simulink model "UIOwDAC_balas_01"  (R2019b)
settings: Solver=VariableStepAuto  StartTime=0.0  StopTime=60  RelTol=1e-3
values from neighbouring files (symbols this model uses):
  A = A-0.1*eye(2)    [DAC_UIO_Comp.m]    (also in LinearND_QUANTUM_2020_11_14_2.m = A+(basis{i}*rand()); UIO_adaptive_example.m = [-2379.2 0 0 0 0;0 -2.3 0 0.21 0; UIO_adaptive_example_2.m = [-1/Ta, (alpha+sigma2*wb2)/Ta, (-kb*sigma2*wb2)/Ta, -kb*sigm; UIO_adaptive_example_EEG_Balas_2ch.m = A-0.4*eye(2))
  Am = double(subs(Am_sys,{ep,Lx},{0.1,1-2*j}))    [DAC_UIO_Comp.m]    (also in UIO_adaptive_example_EEG_Balas_2ch.m = [0 1;-5 -4]; UIO_adaptive_example_alternative_EEG_ch6.m = ss_c.A; UIO_alternative_2021_01_26.m = Am-.1*eye(2); UIO_alternative_PAPER_2021_02_17.m = [0 1;-1 -1])
  B = [0;1]    [DAC_UIO_Comp.m]    (also in UIO_adaptive_example_EEG_Balas_2ch.m; UIO_adaptive_example_alternative_EEG_ch6.m = ones(opt_order,1); UIO_alternative_2021_01_26.m; UIO_alternative_PAPER_2021_02_17.m = [1;0;-1])
  C = double(subs(C_sym,{ep},{0.1}))    [DAC_UIO_Comp.m]    (also in UIO_adaptive_example.m = [1 0 0 0 0;0 0 0 1 0; 0 0 0 0 1]; UIO_adaptive_example_2.m = [1 0 0 0;0 1 0 0]; UIO_adaptive_example_EEG_Balas_2ch.m = [1, epsilon]; UIO_adaptive_example_alternative_EEG_ch6.m = ss_c.C)
  g1 = 4+2j    [DAC_UIO_Comp.m]    (also in UIO_adaptive_example_EEG_Balas_2ch.m = 4; UIO_alternative_2021_01_26.m = 2+1j; UIO_alternative_PAPER_2021_02_17.m = 2; UIO_alternative_PAPER_2021_03_01.m = 2)
  g2 = 0    [DAC_UIO_Comp.m]    (also in UIO_adaptive_example_EEG_Balas_2ch.m = -0.3; UIO_alternative_2021_01_26.m; UIO_alternative_PAPER_2021_02_17.m = 1; UIO_alternative_PAPER_2021_03_01.m)
  g3 = 0    [DAC_UIO_Comp.m]    (also in UIO_adaptive_example_EEG_Balas_2ch.m = 0.1; UIO_alternative_2021_01_26.m; UIO_alternative_PAPER_2021_02_17.m = -3; UIO_alternative_PAPER_2021_03_01.m)
  gamma_e = 1    [DAC_UIO_Comp.m]    (also in UIO_adaptive_example_EEG_Balas_2ch.m; UIO_adaptive_example_alternative_EEG_ch6.m = .0001*ones(length(Am),1); UIO_alternative_2021_01_26.m = 0.001; UIO_alternative_PAPER_2021_02_17.m = 0.0001)
  gamma_u = 1    [DAC_UIO_Comp.m]    (also in UIO_adaptive_example_EEG_Balas_2ch.m = 2)
  sigma_d = 2    [DAC_UIO_Comp.m]
  sigma_e = 1    [DAC_UIO_Comp.m]
settings Model: Creator=Tris  LastModifiedBy=Tris

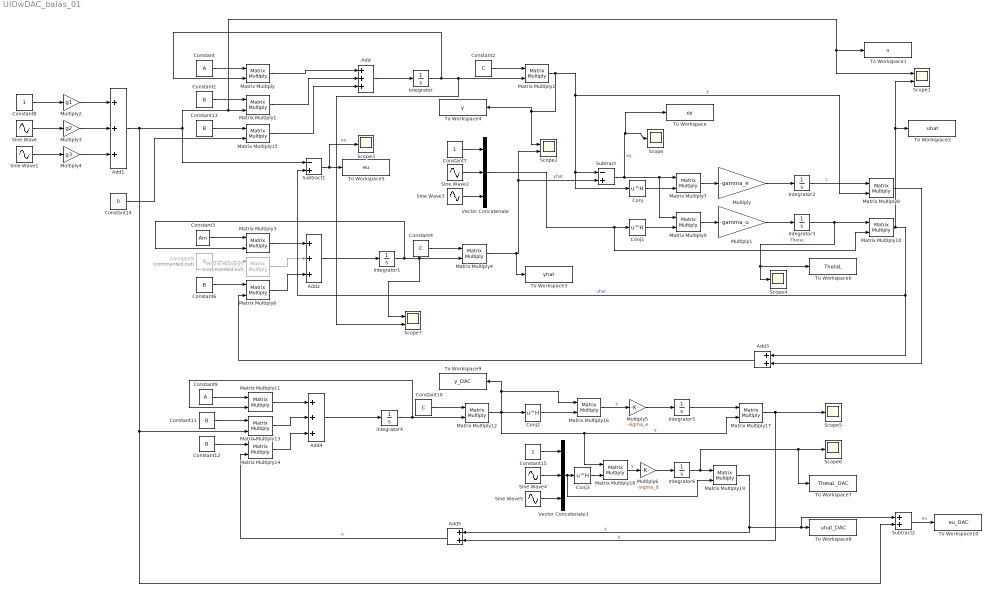
== system UIOwDAC_balas_01 ==
  Add{,1..2,4} (4 alike) : Sum  Inputs=+++
  Add3 : Sum
  Add5 : Sum
  Conj{,1..3} (4 alike) : Math  Operator=hermitian  SignedPower=off  SaturateOnIntegerOverflow=on
  Constant : Constant  Value=A
  Constant{1,6,11..13} (5 alike) : Constant  Value=B  VectorParams1D=off
  Constant10 : Constant  Value=C  VectorParams1D=off
  Constant14 : Constant  Value=0  VectorParams1D=off
  Constant15 : Constant  VectorParams1D=off
  Constant2 : Constant  Value=C  VectorParams1D=off
  Constant3 : Constant  Value=Am
  Constant4 : Constant  Value=C  VectorParams1D=off
  Constant5 : Constant  Commented=on  Value=B  VectorParams1D=off
  Constant7 : Constant  VectorParams1D=off
  Constant8 : Constant  VectorParams1D=off
  Constant9 : Constant  Value=A
  Integrator{,1..6} (7 alike) : Integrator
  Matrix Multiply{,1..4,6..19} (19 alike) : Product  Multiplication=Matrix(*)
  Matrix Multiply5 : Product  Commented=on  Multiplication=Matrix(*)
  Multiply : Gain  Gain=-gamma_e
  Multiply1 : Gain  Gain=-gamma_u
  Multiply2 : Gain  Gain=g1
  Multiply3 : Gain  Gain=g2
  Multiply4 : Gain  Gain=g3
  Multiply5 : Gain  Gain=-sigma_e
  Multiply6 : Gain  Gain=-sigma_d
  Scope{,3..6} (5 alike) : Scope
  Scope1 : Scope  NumInputPorts=2
  Scope2 : Scope  NumInputPorts=2
  Scope7 : Scope  NumInputPorts=2
  Sine Wave : Sin  SampleTime=0  VectorParams1D=off
  Sine Wave1 : Sin  Phase=pi/2  SampleTime=0  VectorParams1D=off
  Sine Wave2 : Sin  SampleTime=0  VectorParams1D=off
  Sine Wave3 : Sin  Phase=pi/2  SampleTime=0  VectorParams1D=off
  Sine Wave4 : Sin  SampleTime=0  VectorParams1D=off
  Sine Wave5 : Sin  Phase=pi/2  SampleTime=0  VectorParams1D=off
  Subtract : Sum  Inputs=-+
  Subtract1 : Sum  Inputs=-+
  Subtract2 : Sum
  To Workspace : ToWorkspace  VariableName=ey  SaveFormat=Timeseries  SampleTime=-1
  To Workspace1 : ToWorkspace  VariableName=u  SaveFormat=Timeseries  SampleTime=-1
  To Workspace10 : ToWorkspace  VariableName=eu_DAC  SaveFormat=Timeseries  SampleTime=-1
  To Workspace2 : ToWorkspace  VariableName=uhat  SaveFormat=Timeseries  SampleTime=-1
  To Workspace3 : ToWorkspace  VariableName=yhat  SaveFormat=Timeseries  SampleTime=-1
  To Workspace4 : ToWorkspace  VariableName=y  SaveFormat=Timeseries  SampleTime=-1
  To Workspace5 : ToWorkspace  VariableName=eu  SaveFormat=Timeseries  SampleTime=-1
  To Workspace6 : ToWorkspace  VariableName=ThetaL  SaveFormat=Timeseries  SampleTime=-1
  To Workspace7 : ToWorkspace  VariableName=ThetaL_DAC  SaveFormat=Timeseries  SampleTime=-1
  To Workspace8 : ToWorkspace  VariableName=uhat_DAC  SaveFormat=Timeseries  SampleTime=-1
  To Workspace9 : ToWorkspace  VariableName=y_DAC  SaveFormat=Timeseries  SampleTime=-1
  Vector Concatenate : Concatenate  NumInputs=3  Mode=Multidimensional array
  Vector Concatenate1 : Concatenate  NumInputs=3  Mode=Multidimensional array
  wires:
  Constant/1 -> Matrix Multiply/1
  Constant1/1 -> Matrix Multiply1/1
  Matrix Multiply/1 -> Add/1
  Matrix Multiply1/1 -> Add/2
  Add/1 -> Integrator/1
  Integrator/1 -> Scope7/2, Matrix Multiply2/2, Matrix Multiply/2
  Constant2/1 -> Matrix Multiply2/1
  Matrix Multiply2/1 -> Scope2/1, To Workspace4/1, Matrix Multiply8/2, Conj/1, Subtract/1  "y"
  Constant8/1 -> Multiply2/1
  Sine Wave/1 -> Multiply3/1
  Sine Wave1/1 -> Multiply4/1
  Add1/1 -> Subtract2/2, Matrix Multiply13/2, Scope1/1, To Workspace1/1, Matrix Multiply1/2, Subtract1/1
  Constant3/1 -> Matrix Multiply3/1
  Matrix Multiply3/1 -> Add2/1
  Add2/1 -> Integrator1/1
  Constant4/1 -> Matrix Multiply4/1
  Integrator1/1 -> Matrix Multiply3/2, Scope7/1, Matrix Multiply4/2
  Matrix Multiply4/1 -> To Workspace3/1, Scope2/2, Subtract/2  "yhat"
  Matrix Multiply5/1 -> Add2/2
  Matrix Multiply6/1 -> Add2/3
  Constant5/1 -> Matrix Multiply5/1
  Constant6/1 -> Matrix Multiply6/1
  Subtract/1 -> To Workspace/1, Scope/1, Matrix Multiply9/1, Matrix Multiply7/1  "ey"
  Conj/1 -> Matrix Multiply7/2
  Matrix Multiply7/1 -> Multiply/1
  Multiply/1 -> Integrator2/1
  Integrator2/1 -> Matrix Multiply8/1  "L"
  Sine Wave3/1 -> Vector Concatenate/3
  Sine Wave2/1 -> Vector Concatenate/2
  Constant7/1 -> Vector Concatenate/1
  Vector Concatenate/1 -> Matrix Multiply10/2, Conj1/1
  Conj1/1 -> Matrix Multiply9/2
  Matrix Multiply9/1 -> Multiply1/1
  Multiply1/1 -> Integrator3/1
  Integrator3/1 -> To Workspace6/1, Scope4/1, Matrix Multiply10/1  "ThetaL"
  Multiply2/1 -> Add1/1
  Multiply3/1 -> Add1/2
  Multiply4/1 -> Add1/3
  Matrix Multiply10/1 -> To Workspace2/1, Scope1/2, Subtract1/2, Add3/1  "uhat"
  Matrix Multiply8/1 -> Add3/2
  Add3/1 -> Matrix Multiply6/2
  Subtract1/1 -> Scope3/1, To Workspace5/1  "eu"
  Matrix Multiply15/1 -> Add/3
  Constant13/1 -> Matrix Multiply15/1
  Constant14/1 -> Matrix Multiply15/2
  Constant9/1 -> Matrix Multiply11/1
  Constant11/1 -> Matrix Multiply13/1
  Constant12/1 -> Matrix Multiply14/1
  Matrix Multiply11/1 -> Add4/1
  Matrix Multiply13/1 -> Add4/2
  Matrix Multiply14/1 -> Add4/3
  Add4/1 -> Integrator4/1
  Integrator4/1 -> Matrix Multiply11/2, Matrix Multiply12/2
  Constant10/1 -> Matrix Multiply12/1
  Matrix Multiply12/1 -> To Workspace9/1, Matrix Multiply16/1, Matrix Multiply18/1, Matrix Multiply17/2, Conj2/1  "y"
  Add5/1 -> Matrix Multiply14/2  "u"
  Conj2/1 -> Matrix Multiply16/2
  Matrix Multiply16/1 -> Multiply5/1  "y"
  Multiply5/1 -> Integrator5/1
  Integrator5/1 -> Matrix Multiply17/1
  Matrix Multiply17/1 -> Scope5/1, Add5/2  "y"
  Constant15/1 -> Vector Concatenate1/1
  Sine Wave5/1 -> Vector Concatenate1/3
  Sine Wave4/1 -> Vector Concatenate1/2
  Vector Concatenate1/1 -> Matrix Multiply19/2, Conj3/1
  Conj3/1 -> Matrix Multiply18/2
  Matrix Multiply18/1 -> Multiply6/1  "y"
  Multiply6/1 -> Integrator6/1
  Integrator6/1 -> To Workspace7/1, Scope6/1, Matrix Multiply19/1
  Matrix Multiply19/1 -> Subtract2/1, To Workspace8/1, Add5/1  "y"
  Subtract2/1 -> To Workspace10/1  "eu"
